simulink model "plutoradiofreqcalib_rx"  (R2021a)
settings: Solver=FixedStepDiscrete  StartTime=0.0  StopTime=inf  RelTol=1e-3  EnableMultiTasking=on
undefined symbols (not defined in the file): Fs, ip, usb
libraries: plutoradiolib x1, dspspect3 x1
settings Model: Creator=The MathWorks, Inc.  LastModifiedBy=Bornitz
settings SolverCC: AlgebraicLoopSolver=TrustRegion
settings DataIOCC: LimitDataPoints=on  SaveFormat=Array  ReturnWorkspaceOutputs=off
settings OptimizationCC: ExpressionDepthLimit=2147483647  LifeSpan=inf
settings DebuggingCC: UnderspecifiedInitializationDetection=Classic  MergeDetectMultiDrivingBlocksExec=none  SolverPrmCheckMsg=warning  ParameterPrecisionLossMsg=none  FcnCallInpInsideContextMsg=warning  AllowSymbolicDim=off  StateNameClashWarn=warning  SFUnexpectedBacktrackingDiag=warning  SFNoUnconditionalDefaultTransitionDiag=warning  SFExecutionAtInitializationDiag=none  SFMachineParentedDataDiag=warning  ArithmeticOperatorsInVariantConditions=warning
settings HardwareCC: ProdBitPerPointer=32  ProdBitPerSizeT=32  ProdBitPerPtrDiffT=32  ProdLargestAtomicFloat=None  ProdIntDivRoundTo=Undefined  ProdEndianess=Unspecified  ProdWordSize=32  ProdHWDeviceType=32-bit Generic  TargetBitPerPointer=64  TargetBitPerSizeT=64  TargetBitPerPtrDiffT=64  TargetLongLongMode=on  TargetIntDivRoundTo=Zero  TargetEndianess=LittleEndian  TargetWordSize=64  TargetHWDeviceType=Generic->MATLAB Host Computer  ProdEqTarget=off
settings ModelReferenceCC: PropagateSignalLabelsOutOfModel=off
settings SFSimCC: SimUseLocalCustomCode=off  CustomCodeUndefinedFunction=UseInterfaceOnly
settings RTWCC: RTWUseLocalCustomCode=off
settings RTWCC: CustomSourceCode=|
  | #include<stdio.h>
  | #include<stdlib.h>
settings CodeAppCC: StateflowObjectComments=on
settings GRTTargetCC: TargetLangStandard=C89/C90 (ANSI)  CombineOutputUpdateFcns=off  GRTInterface=on
settings ConfigComp: CovMetricSettings=dw  CovSaveCumulativeToWorkspaceVar=on  CovSaveSingleToWorkspaceVar=on  CovExternalEMLEnable=off  CovSFcnEnable=off

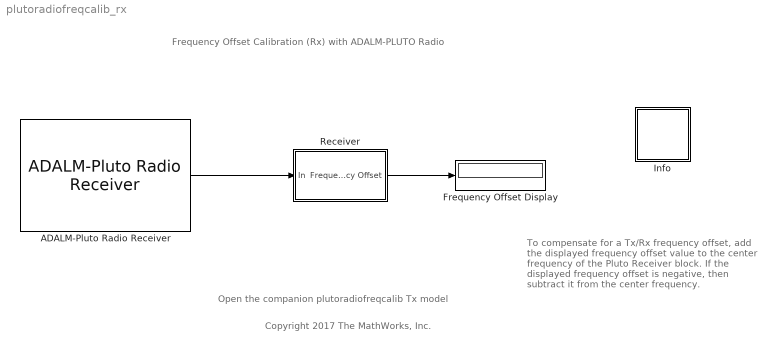
== system plutoradiofreqcalib_rx ==
  note: Frequency Offset Calibration (Rx)
      | with ADALM-PLUTO Radio
  note: Open the companion plutoradiofreqcalib Tx model
  note: Copyright 2017 The MathWorks, Inc.
  note: To compensate for a Tx/Rx frequency offset,
      | add the displayed frequency offset value to the
      | center frequency of the Pluto Receiver block. If
      | the displayed frequency offset is negative, then
      | subtract it from the center frequency.
  ADALM-Pluto Radio Receiver : plutoradiolib/ADALM-Pluto Radio Receiver  RadioID=usb:0  uri=ip:10.0.0.200  CenterFrequencySource=Dialog  CenterFrequency=1.85e9  GainSource=AGC Fast Attack  GainSourceBlock=AGC Slow Attack  Gain=20  ChannelMapping=1  BasebandSampleRate=100e3  OutputDataType=double  SamplesPerFrame=10000  OverflowOutputPort=off  EnableBurstMode=off  NumFramesInBurst=1  ShowAdvancedProperties=off  UseCustomFilter=off  filtPathRates=[737280000 11520000 3840000 1920000 960000 240000]  filtCoefficients=[-192 82 85 -215 228 -102 -110 290 -318 145 160 -426 471 -215 -238 633 -697 318 349 -923 1009 -457 -498 1309 -1423 640 693 -1812 1959 -876 -945 2458 -2647 1180 1268 -3290 3534 -1572 -1688 4375 -4698 2091 2247 -5836 6284 -2807 -3031 7918 -8588 3870 4225 -11182 12324 -5662 -6330 17255 -19735 9507 11312 -33568 43355 -25227 -42139 305542 305542 -42139 -25227 43355 -33568 11312 9507 -19735 17255 -6330 -5662 12324 -11182 4225 3870 -8588 7918 -3031 -2807 6284 -5836 2247 2091 -4698 4375 -1688 -1572 3534 -3290 1268 1180 -2647 2458 -945 -876 1959 -1812 693 640 -1423 1309 -498 -457 1009 -923 349 318 -697 633 -238 -215 471 -426 160 145 -318 290 -110 -102 228 -215 85 82 -192]  filtCoefficientSize=128  filtDecimInterpFactor=4  filtGain=-12  filtRFBandwidth=18000000  filterConfigStruct=struct()  EnableQuadratureCorrection=on  EnableRFDCCorrection=on  EnableBasebandDCCorrection=on  FrequencyCorrection=0  OverrideSampleTime=off  SampleTime=0.02  DataTimeout=Inf  ENSMPinControlMode=None  BISTLoopbackMode=Disabled  BISTToneInject=Disabled  BISTSignalGen=PRBS  BISTToneFreq=Fs/32  BISTToneLevel=0
      settings: SourceProductBaseCode=PLUTO
  Frequency Offset Display : Display
  Info : Subsystem  LoadFcn=plutoradiosetup  mask(Info){}
      settings: OpenFcn=plutoradiodoc('plutoradiofreqcalib');
      mask Display: disp('Info')
  Receiver : Subsystem
      mask Display: disp('Receiver')
  wires:
  Receiver/1(Frequency Offset) -> Frequency Offset Display/1
  ADALM-Pluto Radio Receiver/1 -> Receiver/1(In)

== system plutoradiofreqcalib_rx/Info ==

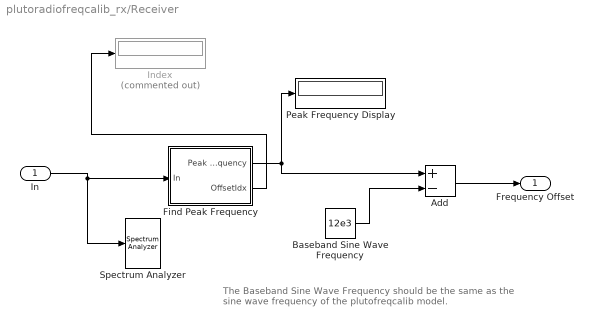
== system plutoradiofreqcalib_rx/Receiver ==
  note: The Baseband Sine Wave Frequency should be the same as
      | the sine wave frequency of the plutofreqcalib model.
  In : Inport
  Add : Sum  Inputs=+-
  Baseband Sine Wave Frequency : Constant  Value=12e3
  Find Peak Frequency : Subsystem
      mask Display: disp('Find Peak\nFrequency')
  Index : Display  Commented=on
  Peak Frequency Display : Display
  Spectrum Analyzer : SpectrumAnalyzer
  Frequency Offset : Outport  VectorParamsAs1DForOutWhenUnconnected=off
  wires:
  Baseband Sine Wave Frequency/1 -> Add/2
  Add/1 -> Frequency Offset/1
  In/1 -> Spectrum Analyzer/1, Find Peak Frequency/1(In)
  Find Peak Frequency/1(Peak Frequency) -> Add/1, Peak Frequency Display/1
  Find Peak Frequency/2(OffsetIdx) -> Index/1

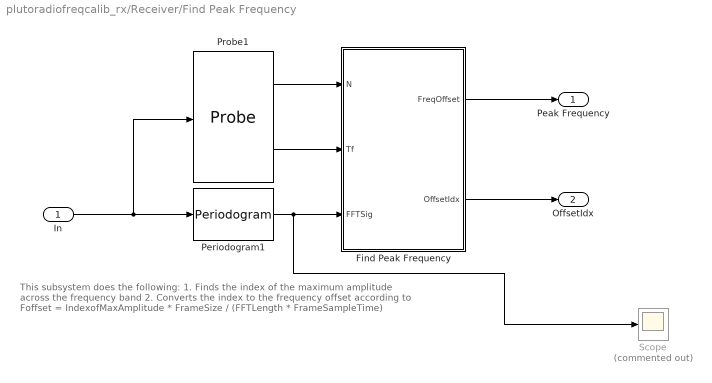
== system plutoradiofreqcalib_rx/Receiver/Find Peak Frequency ==
  note: This subsystem does the following:
      | 1.  Finds the index of the maximum amplitude across the frequency band
      | 2.  Converts the index to the frequency offset according to
      | Foffset = IndexofMaxAmplitude * FrameSize / (FFTLength * FrameSampleTime)
  In : Inport
  Find Peak Frequency : MATLAB Function  TreatAsAtomicUnit=on
  Periodogram1 : dspspect3/Periodogram  measurement=Power spectral density  wintype=Hamming  Rs=50  beta=5  winsamp=Symmetric  FFTImplementation=Auto  inheritFFT=off  fftsize=2048  navg=2  inheritTs=on  Ts=1
      settings: SourceProductBaseCode=DS
  Probe1 : Probe  ProbeComplexSignal=off
  Scope : Scope  Commented=on
  Peak Frequency : Outport  VectorParamsAs1DForOutWhenUnconnected=off
  OffsetIdx : Outport  Port=2  VectorParamsAs1DForOutWhenUnconnected=off
  wires:
  Periodogram1/1 -> Scope/1, Find Peak Frequency/3(FFTSig)
  Probe1/1 -> Find Peak Frequency/1(N)
  Probe1/2 -> Find Peak Frequency/2(Tf)
  Find Peak Frequency/1(FreqOffset) -> Peak Frequency/1
  In/1 -> Periodogram1/1, Probe1/1
  Find Peak Frequency/2(OffsetIdx) -> OffsetIdx/1

== matlab function plutoradiofreqcalib_rx/Receiver/Find Peak Frequency/Find Peak Frequency ==
  data: N input; FreqOffset output; Tf input; FFTSig input; OffsetIdx output
function  [FreqOffset, OffsetIdx] = findpeakfreq(N, Tf, FFTSig)
% Find peak frequency
% N - frame size
% Tf - frame sample time
% FFTSig - result of FFT

%#codegen

FFTSize = length(FFTSig);
FFTSig = fftshift(FFTSig);
[~, maxIdx] = max(FFTSig); % Find index of max magnitude
OffsetIdx = maxIdx-1-FFTSize/2; % Convert to index symmetric with 0
% probably mistaking if negative freq is max
% resolution df round 48Hz 
Ts = Tf(1)/N; % Sample time
delta_f = 1/Ts/FFTSize; % Frequency resolution of FFT
FreqOffset = OffsetIdx*delta_f;% Map offset index back to frequency
